simulink model "LCL_SIM"  (R2022a)
settings: Solver=VariableStepAuto  StartTime=0.0  StopTime=0.02*8  FixedStep=Ts  RelTol=1e-3
values from neighbouring files (symbols this model uses):
  C = 10e-06    (= 1e-05)    [LCL_Filter_Analysis.m]    (also in Lowpass_Filer_Design.m = tf(num_c,den_c,Ts); Parameter.m)
  L1 = 600e-06    (= 0.0006)    [LCL_Filter_Analysis.m]    (also in Lowpass_Filer_Design.m; Parameter.m)
  R = 2    [LCL_Filter_Analysis.m]    (also in Lowpass_Filer_Design.m = 1.5; Parameter.m = 1.5)
  Ts = 0.02/800    (= 2.5e-05)    [Lowpass_Filer_Design.m]    (also in Parameter.m)
  Vin = 360    [Parameter.m]
  Vtri = 3.05    [Parameter.m]
libraries: spsACVoltageSourceLib x9, spsIGBTDiodeLib x4, spsSeriesRLCBranchLib x3, spsCurrentMeasurementLib x3, spsVoltageMeasurementLib x2, spsDCVoltageSourceLib x1, spsGroundLib x1, simulink x1, slpidlib x1, spsTriangleGeneratorLib x1, spsPLLLib x1, spspowerguiLib x1
settings Model: Creator=hoang  LastModifiedBy=hoanghua
settings SolverCC: ZeroCrossAlgorithm=Adaptive  AlgebraicLoopSolver=TrustRegion
settings DataIOCC: ReturnWorkspaceOutputs=off
settings DebuggingCC: IgnoredZcDiagnostic=none  UnconnectedInputMsg=warning  UnconnectedOutputMsg=warning  UnconnectedLineMsg=warning  SFMachineParentedDataDiag=warning

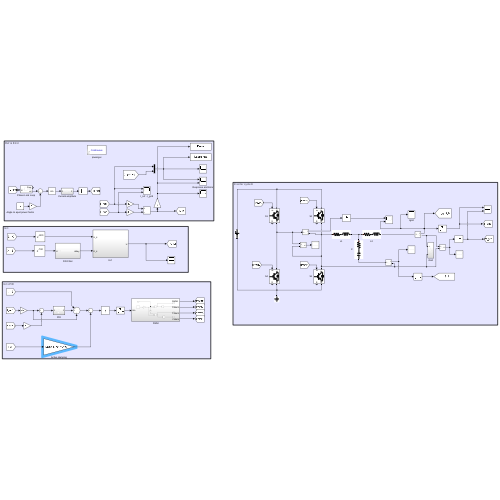
[thumbnail: Simulink's stored preview of the top-level diagram]
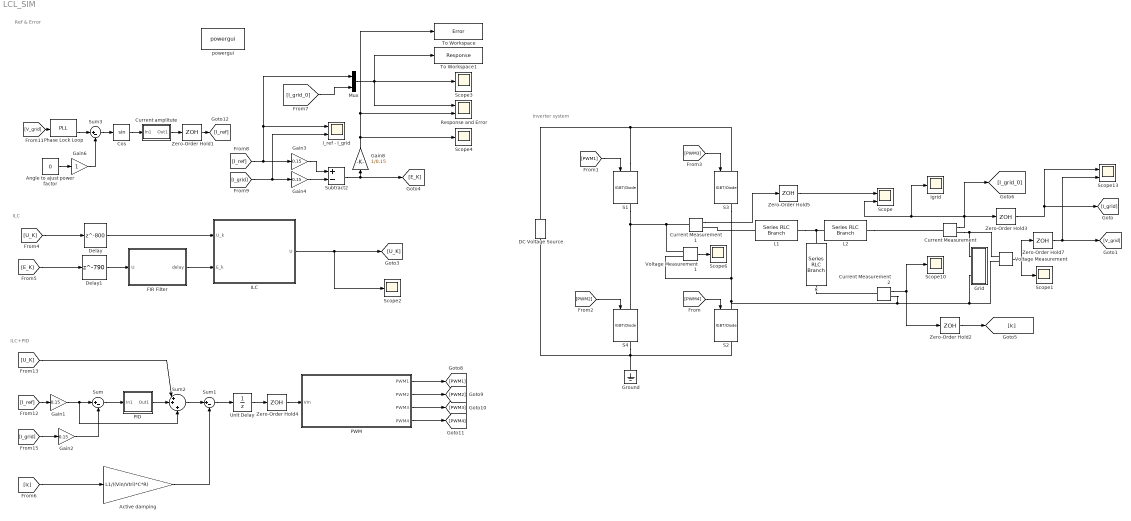
== system LCL_SIM ==
  note: ILC+PID
  note: Inverter system
  note: Ref & Error
  note: ILC
  Active damping : Gain  Gain=L1/((Vin/Vtri)*C*R)
  Angle to ajust power factor : Constant  Value=0
  C : spsSeriesRLCBranchLib/Series RLC Branch  LConnTagsString=__new0  RConnTagsString=__new0  BranchType=RC  Resistance=0.00  Inductance=600e-6  SetiL0=off  InitialCurrent=0  Capacitance=10e-6  Setx0=off  InitialVoltage=0  Measurements=None
  Cos : Trigonometry
  Current Measurement : spsCurrentMeasurementLib/Current Measurement  PhasorSimulation=off  OutputType=Complex  PSBequivalent=0
  Current Measurement1 : spsCurrentMeasurementLib/Current Measurement  PhasorSimulation=off  OutputType=Complex  PSBequivalent=0
  Current Measurement2 : spsCurrentMeasurementLib/Current Measurement  PhasorSimulation=off  OutputType=Magnitude  PSBequivalent=0
  Current amplitute : Subsystem
  DC Voltage Source : spsDCVoltageSourceLib/DC Voltage Source  Amplitude=360  Measurements=None
  Delay : Delay  DelayLength=800  SampleTime=Ts
  Delay1 : Delay  DelayLength=790  SampleTime=Ts
  FIR Filter : Subsystem
  Gain{1..4} (4 alike) : Gain  Gain=0.15
  Gain6 : Gain
  Gain8 : Gain  Gain=1/0.15
  Grid : Subsystem
  Ground : spsGroundLib/Ground  LConnTagsString=a
  "ILC " : Subsystem
  I_ref - I_grid : Scope  NumInputPorts=2
  Igrid : Scope
  L1 : spsSeriesRLCBranchLib/Series RLC Branch  LConnTagsString=__new0  RConnTagsString=__new0  BranchType=RL  Resistance=0  Inductance=600e-6  SetiL0=on  InitialCurrent=0  Capacitance=0  Setx0=off  InitialVoltage=0  Measurements=None
  L2 : spsSeriesRLCBranchLib/Series RLC Branch  LConnTagsString=__new0  RConnTagsString=__new0  BranchType=RL  Resistance=0  Inductance=150e-6  SetiL0=on  InitialCurrent=0  Capacitance=0  Setx0=off  InitialVoltage=0  Measurements=None
  Mux : Mux  Inputs=2
  PID : Subsystem
  PWM : Subsystem
  Phase Lock Loop : spsPLLLib/PLL  Fmin=45  Par_Init=[0, 50.1]  ParK=[180, 3200, 1]  TcD=1e-4  MaxRateChangeFreq=12  FilterCutOffFreq=25  Ts=0  AGC=on
      settings: SourceProductBaseCode=PS
  Response and Error : Scope  NumInputPorts=2
  S{1..4} (4 alike) : spsIGBTDiodeLib/IGBT//Diode  Ron=1e-3  Rs=1e5  Cs=inf  Measurements=on
  Scope : Scope  NumInputPorts=2
  Scope{1..4,6,10} (6 alike) : Scope
  Scope13 : Scope  NumInputPorts=2
  Subtract2 : Sum  Inputs=+-
  Sum : Sum  Inputs=|+-
  Sum1 : Sum  Inputs=|+-
  Sum2 : Sum  Inputs=|++|+
  Sum3 : Sum  Inputs=|+-
  To Workspace : ToWorkspace  VariableName=Error  SaveFormat=Timeseries  SampleTime=Ts
  To Workspace1 : ToWorkspace  VariableName=Response  SaveFormat=Timeseries  SampleTime=Ts
  Unit Delay : UnitDelay  SampleTime=-1  HasFrameUpgradeWarning=on
  Voltage Measurement : spsVoltageMeasurementLib/Voltage Measurement  PhasorSimulation=off  OutputType=Complex  PSBequivalent=0
  Voltage Measurement1 : spsVoltageMeasurementLib/Voltage Measurement  PhasorSimulation=off  OutputType=Complex  PSBequivalent=0
  Zero-Order Hold{1,3,5,7} (4 alike) : ZeroOrderHold  SampleTime=Ts
  Zero-Order Hold2 : ZeroOrderHold  SampleTime=Ts/100
  Zero-Order Hold4 : ZeroOrderHold  SampleTime=Ts/100
  powergui : spspowerguiLib/powergui  Priority=1  SimulationMode=Continuous  SampleTime=0.02/500  frequency=50  Iterations=50  frequencyindice=50  Pbase=100e6  ErrMax=1e-4  UnitsV=kV  UnitsW=MW  buscounter=0  FunctionMessages=on  echomessages=off  EnableUseOfTLC=off  CurrentSourceSwitches=off  DisableSnubberDevices=off  DisableRonSwitches=off  DisableVfSwitches=off  DisplayEquations=off  AutomaticDiscreteSolvers=off  SolverType=Tustin/Backward Euler (TBE)  Interpol=off  ExternalGateDelay=off  methode=off  Ts=100  x0status=blocks  SPID=off  SwTol=0  HookPort=off  NonlinearTolerance=1e-4  nMaxIteration=100  ContinueOnMaxIteration=off  RestoreLinks=warning  ResistiveCurrentMeasurement=off  Frange=[0:2:500]  Ylog=off  Xlog=on  ShowGrid=off  save=off  variable=ZData  structure=Igrid  ZoomFFT=off  StartTime=0.1  cycles=3  DisplayStyle=2  fundamental=50  FreqAxis=on  MaxFrequency=3000  frequencyindicesteady=1  RmsSteady=1  display=off
  wires:
  Gain4/1 -> Subtract2/2
  [E_K] -> Delay1/1
  [U_K] -> Delay/1
  [I_grid] -> I_ref - I_grid/2, Gain4/1
  Subtract2/1 -> Gain8/1, [E_K]
  "ILC "/1(U) -> [U_K], Scope2/1
  [I_ref] -> Mux/1, I_ref - I_grid/1, Gain3/1
  [V_grid] -> Phase Lock Loop/1
  [I_grid_0] -> Mux/2
  Mux/1 -> Scope3/1, To Workspace1/1, Response and Error/1
  Angle to ajust power factor/1 -> Gain6/1
  Phase Lock Loop/2 -> Sum3/1
  Gain6/1 -> Sum3/2
  Sum3/1 -> Cos/1
  Cos/1 -> Current amplitute/1(In1)
  Gain8/1 -> To Workspace/1, Response and Error/2, Scope4/1
  Gain3/1 -> Subtract2/1
  Delay/1 -> "ILC "/1(U_k)
  FIR Filter/1(delay) -> "ILC "/2(E_k)
  Delay1/1 -> FIR Filter/1(U)
  Current amplitute/1(Out1) -> Zero-Order Hold1/1
  Zero-Order Hold1/1 -> [I_ref]
  Voltage Measurement/1 -> Scope1/1, Zero-Order Hold7/1
  Current Measurement2/1 -> Zero-Order Hold2/1, Scope10/1
  [PWM2] -> S4/1
  Current Measurement1/1 -> Zero-Order Hold5/1
  Current Measurement/1 -> [I_grid_0], Igrid/1, Scope/2, Zero-Order Hold3/1
  [PWM3] -> S3/1
  Zero-Order Hold2/1 -> [Ic]
  Zero-Order Hold3/1 -> Scope13/1, [I_grid]
  Voltage Measurement1/1 -> Scope6/1
  Zero-Order Hold7/1 -> Scope13/2, [V_grid]
  [PWM1] -> S1/1
  Zero-Order Hold5/1 -> Scope/1
  [PWM4] -> S2/1
  PWM/1("PWM1 ") -> [PWM1]
  Zero-Order Hold4/1 -> PWM/1(Vm)
  PWM/4(PWM4) -> [PWM4]
  Active damping/1 -> Sum1/2
  Gain2/1 -> Sum/2
  [U_K] -> Sum2/1
  Sum/1 -> PID/1(In1)
  Sum1/1 -> Unit Delay/1
  Sum2/1 -> Sum1/1
  Unit Delay/1 -> Zero-Order Hold4/1
  PWM/3(PWM3) -> [PWM3]
  [I_ref] -> Gain1/1
  PWM/2(PWM2) -> [PWM2]
  [Ic] -> Active damping/1
  Gain1/1 -> Sum/1, Sum2/3
  [I_grid] -> Gain2/1
  PID/1(Out1) -> Sum2/2
  connections:
  C/RConn1 -- Current Measurement2/LConn1
  Current Measurement/RConn1 -- Voltage Measurement/LConn1 -- Grid/LConn1
  S1/LConn1 -- S3/LConn1 -- DC Voltage Source/RConn1
  S3/RConn1 -- Current Measurement2/RConn1 -- Voltage Measurement/LConn2 -- Grid/LConn2 -- S2/LConn1 -- Voltage Measurement1/LConn2
  DC Voltage Source/LConn1 -- S4/RConn1 -- S2/RConn1 -- Ground/LConn1
  Current Measurement1/LConn1 -- S4/LConn1 -- S1/RConn1 -- Voltage Measurement1/LConn1
  L1/LConn1 -- Current Measurement1/RConn1
  C/LConn1 -- L2/LConn1 -- L1/RConn1
  L2/RConn1 -- Current Measurement/LConn1

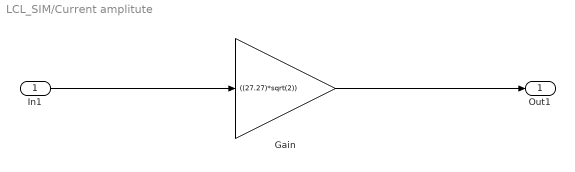
== system LCL_SIM/Current amplitute ==
  In1 : Inport
  Gain : Gain  Gain=((27.27)*sqrt(2))
  Out1 : Outport
  wires:
  In1/1 -> Gain/1
  Gain/1 -> Out1/1

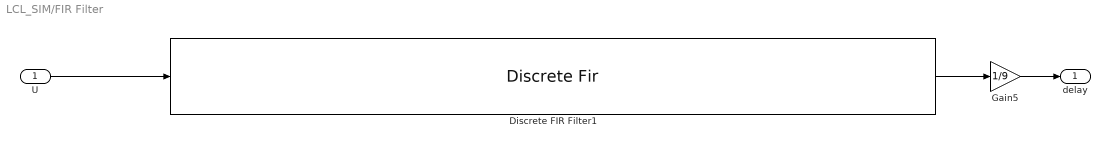
== system LCL_SIM/FIR Filter ==
  U : Inport
  Discrete FIR Filter1 : DiscreteFir  Coefficients=[1 1 1 1 1 1 1 1 1]  SampleTime=Ts
  Gain5 : Gain  Gain=1/9
  delay : Outport  VectorParamsAs1DForOutWhenUnconnected=off
  wires:
  Gain5/1 -> delay/1
  Discrete FIR Filter1/1 -> Gain5/1
  U/1 -> Discrete FIR Filter1/1

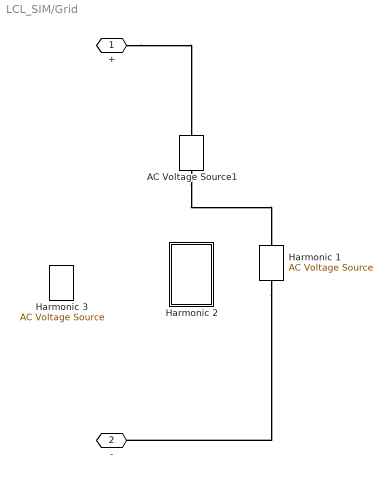
== system LCL_SIM/Grid ==
  AC Voltage Source1 : spsACVoltageSourceLib/AC Voltage Source  Amplitude=220*sqrt(2)  Phase=0  Frequency=50  SampleTime=0  Measurements=None  BusType=PV  Pref=6e3  Qref=0  Qmin=-inf  Qmax=+inf
  Harmonic 1 : spsACVoltageSourceLib/AC Voltage Source  Amplitude=220*sqrt(2)*0.01  Phase=0  Frequency=50*33  SampleTime=0  Measurements=None  BusType=PV  Pref=6e3  Qref=0  Qmin=-inf  Qmax=+inf
  Harmonic 2 : Subsystem
      settings: PortSchema="{\"entries\":[{\"content\":{\"sides\":[{\"content\":{\"connectorIds\":[]},\"type\":\"ConnectorPlacement.EquallySpacedRectSide\",\"uuid\":\"f60a8588-046c-4c4f-94c2-27eb35b2c768\"},{\"content\":{\"connectorIds\":[],\"side\":\"RIGHT\"},\"type\":\"ConnectorPlacement.EquallySpacedRectSide\",\"uuid\":\"a6fd0e6d-caa2-4954-9545-666586426112\"},{\"content\":{\"connectorIds\":[\"LConn1\"],\"side\":\"TOP\"},\"type\":\"ConnectorPlacement.EquallySpacedRectSide\",\"uuid\":\"3887d386-67a4-4090-b26b-c77f8cd89017\"},{\"content\":{\"connectorIds\":[\"RConn1\"],\"side\":\"BOTTOM\"},\"type\":\"ConnectorPlacement.EquallySpacedRectSide\",\"uuid\":\"506826a6-9c45-4d5d-96d6-c56dbc9a3480\"}]},\"type\":\"ConnectorPlacement.EquallySpacedConnector\",\"uuid\":\"c15ad883-a9a3-491e-b546-5f76a0de8772\"}],\"packageUris\":[\"http://schema.mathworks.com/mf0/Connector/19700101\"],\"version\":\"1.0\"}"
  Harmonic 3 : spsACVoltageSourceLib/AC Voltage Source  Amplitude=220*sqrt(2)*0.1  Phase=0  Frequency=50*3  SampleTime=0  Measurements=None  BusType=PV  Pref=6e3  Qref=0  Qmin=-inf  Qmax=+inf
  + : PMIOPort  Side=Left
  - : PMIOPort  Port=2  Side=Left
  connections:
  +/RConn1 -- AC Voltage Source1/RConn1
  AC Voltage Source1/LConn1 -- Harmonic 1/RConn1
  Harmonic 1/LConn1 -- -/RConn1

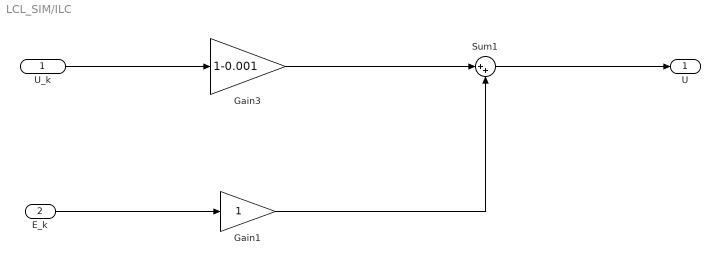
== system LCL_SIM/ILC  ==
  U_k : Inport
  E_k : Inport  Port=2
  Gain1 : Gain
  Gain3 : Gain  Gain=1-0.001
  Sum1 : Sum  Inputs=|++
  U : Outport  VectorParamsAs1DForOutWhenUnconnected=off
  wires:
  U_k/1 -> Gain3/1
  Sum1/1 -> U/1
  E_k/1 -> Gain1/1
  Gain3/1 -> Sum1/1
  Gain1/1 -> Sum1/2

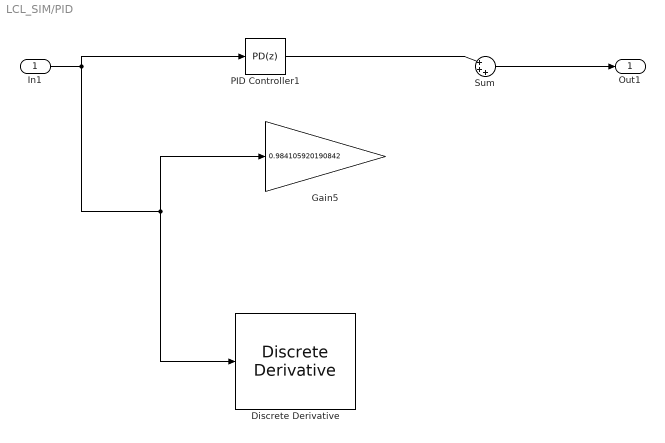
== system LCL_SIM/PID ==
  In1 : Inport
  Discrete Derivative : simulink/Discrete/Discrete Derivative  gainval=6.59449920156203e-05  ICPrevScaledInput=0.0  OutMin=[]  OutMax=[]  OutDataType=fixdt(1, 16)  OutScaling=2^-10  DoSatur=off
  Gain5 : Gain  Gain=0.984105920190842
  PID Controller1 : slpidlib/PID Controller  Controller=PD  Form=Parallel  TimeDomain=Discrete-time  UseExternalTs=off  SampleTime=Ts  IntegratorMethod=Forward Euler  FilterMethod=Forward Euler  ControllerParametersSource=internal  P=0.984105920190842  I=2200  UseKiTs=off  D=6.59449920156203e-05  N=10000000000000000  UseFilter=off  TunerSelectOption=Transfer Function Based (PID Tuner App)  InitialConditionSource=internal  InitialConditionForIntegrator=0  InitialConditionForFilter=0  DifferentiatorICPrevScaledInput=0  ExternalReset=none  TrackingMode=off  Kt=1  LimitOutput=off  SatLimitsSource=internal  UpperSaturationLimit=inf  LowerSaturationLimit=-inf  LinearizeAsGain=on  AntiWindupMode=none  Kb=1  POutMin=[]  POutMax=[]  IOutMin=[]  IOutMax=[]  DOutMin=[]  DOutMax=[]  NOutMin=[]  NOutMax=[]  SumOutMin=[]  SumOutMax=[]  SaturationOutMin=[]  SaturationOutMax=[]  PParamMin=[]  PParamMax=[]  IParamMin=[]  IParamMax=[]  DParamMin=[]  DParamMax=[]  NParamMin=[]  NParamMax=[]  KbParamMin=[]  KbParamMax=[]  KtParamMin=[]  KtParamMax=[]  KbOutMin=[]  KbOutMax=[]  KtOutMin=[]  KtOutMax=[]  IntegratorOutMin=[]  IntegratorOutMax=[]  FilterOutMin=[]  FilterOutMax=[]  SumI1OutMin=[]  SumI1OutMax=[]  SumI2OutMin=[]  SumI2OutMax=[]  SumI3OutMin=[]  SumI3OutMax=[]  SumI4OutMin=[]  SumI4OutMax=[]  SumDOutMin=[]  SumDOutMax=[]  DifferentiatorOutMin=[]  DifferentiatorOutMax=[]  FilterDiffOutCoefMin=[]  FilterDiffOutCoefMax=[]  ReciprocalOutMin=[]  ReciprocalOutMax=[]  SumDenOutMin=[]  SumDenOutMax=[]  SumNumOutMin=[]  SumNumOutMax=[]  DivideOutMin=[]  DivideOutMax=[]  UdiffTsProdOutMin=[]  UdiffTsProdOutMax=[]  NTsProdOutMin=[]  NTsProdOutMax=[]  UintegralTsProdOutMin=[]  UintegralTsProdOutMax=[]  UngainTsProdOutMin=[]  UngainTsProdOutMax=[]  IntegratorContinuousStateAttributes=''  IntegratorStateMustResolveToSignalObject=off  IntegratorRTWStateStorageClass=Auto  FilterContinuousStateAttributes=''  FilterStateMustResolveToSignalObject=off  FilterRTWStateStorageClass=Auto  ParallelPVariant=InternalParameters  IdealPVariant=Disabled  IVariant=Disabled  DVariant=InternalParameters  IntegratorVariant=Disabled  SatVariant=Disabled  AWVariant=Disabled  PCopyVariant=Disabled  TRVariant=Disabled  FdbkBlocksVariant=Forward  IdealPFdbkVariant=Disabled  SatFdbkVariant=Disabled  DerivativeFilterVariant=Differentiator  NVariant=Passthrough  NCopyVariant=Disabled_SignalSpec  FilterICVariant=InternalICsDifferentiator  IntegratorICVariant=Disabled  ExternalResetVariant=Disabled  TRSumVariant=Passthrough  SumFdbkVariant=Disabled  SumVariant=Sum_PD  TsampFilterVariant=InternalTs  TsampNgainVariant=Passthrough  TsampIntegralVariant=Disabled_SignalSpec  ExternalSaturationOutDataTypeStr=Inherit: Same as second input  aMode=0
  Sum : Sum  Inputs=|+++
  Out1 : Outport  VectorParamsAs1DForOutWhenUnconnected=off
  wires:
  Sum/1 -> Out1/1
  In1/1 -> PID Controller1/1, Discrete Derivative/1, Gain5/1
  PID Controller1/1 -> Sum/1

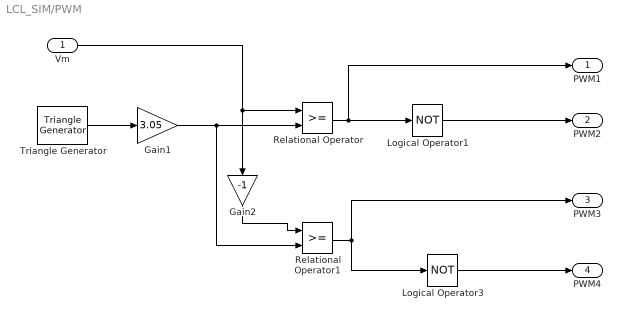
== system LCL_SIM/PWM ==
  Vm : Inport
  Gain1 : Gain  Gain=3.05
  Gain2 : Gain  Gain=-1
  Logical Operator1 : Logic  Operator=NOT  AllPortsSameDT=off  OutDataTypeStr=boolean
  Logical Operator3 : Logic  Operator=NOT  AllPortsSameDT=off  OutDataTypeStr=boolean
  Relational Operator : RelationalOperator  OutDataTypeStr=boolean  RndMeth=Simplest  InputSameDT=off
  Relational Operator1 : RelationalOperator  OutDataTypeStr=boolean  RndMeth=Simplest  InputSameDT=off
  Triangle Generator : spsTriangleGeneratorLib/Triangle Generator  Freq=10e3  Phase=0  Ts=0
  "PWM1 " : Outport  VectorParamsAs1DForOutWhenUnconnected=off
  PWM2 : Outport  Port=2  VectorParamsAs1DForOutWhenUnconnected=off
  PWM3 : Outport  Port=3  VectorParamsAs1DForOutWhenUnconnected=off
  PWM4 : Outport  Port=4  VectorParamsAs1DForOutWhenUnconnected=off
  wires:
  Vm/1 -> Gain2/1, Relational Operator/1
  Triangle Generator/1 -> Gain1/1
  Gain1/1 -> Relational Operator1/2, Relational Operator/2
  Relational Operator/1 -> "PWM1 "/1, Logical Operator1/1
  Logical Operator1/1 -> PWM2/1
  Relational Operator1/1 -> PWM3/1, Logical Operator3/1
  Gain2/1 -> Relational Operator1/1
  Logical Operator3/1 -> PWM4/1

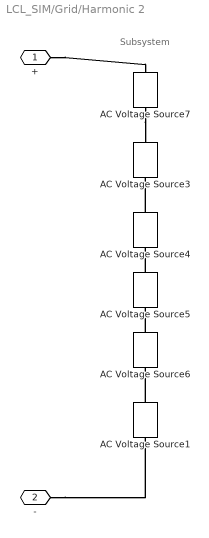
== system LCL_SIM/Grid/Harmonic 2 ==
  note: Subsystem
  AC Voltage Source1 : spsACVoltageSourceLib/AC Voltage Source  Amplitude=220*sqrt(2)*0.02  Phase=0  Frequency=50*13  SampleTime=0  Measurements=None  BusType=PV  Pref=6e3  Qref=0  Qmin=-inf  Qmax=+inf
  AC Voltage Source3 : spsACVoltageSourceLib/AC Voltage Source  Amplitude=220*sqrt(2)*0.05  Phase=90  Frequency=50*5  SampleTime=0  Measurements=None  BusType=PV  Pref=6e3  Qref=0  Qmin=-inf  Qmax=+inf
  AC Voltage Source4 : spsACVoltageSourceLib/AC Voltage Source  Amplitude=220*sqrt(2)*0.03  Phase=0  Frequency=50*7  SampleTime=0  Measurements=None  BusType=PV  Pref=6e3  Qref=0  Qmin=-inf  Qmax=+inf
  AC Voltage Source5 : spsACVoltageSourceLib/AC Voltage Source  Amplitude=220*sqrt(2)*0.03  Phase=0  Frequency=50*9  SampleTime=0  Measurements=None  BusType=PV  Pref=6e3  Qref=0  Qmin=-inf  Qmax=+inf
  AC Voltage Source6 : spsACVoltageSourceLib/AC Voltage Source  Amplitude=220*sqrt(2)*0.02  Phase=0  Frequency=50*11  SampleTime=0  Measurements=None  BusType=PV  Pref=6e3  Qref=0  Qmin=-inf  Qmax=+inf
  AC Voltage Source7 : spsACVoltageSourceLib/AC Voltage Source  Amplitude=220*sqrt(2)*0.1  Phase=0  Frequency=50*3  SampleTime=0  Measurements=None  BusType=PV  Pref=6e3  Qref=0  Qmin=-inf  Qmax=+inf
  + : PMIOPort  Side=Left
  - : PMIOPort  Port=2  Side=Right
  connections:
  AC Voltage Source7/LConn1 -- AC Voltage Source3/RConn1
  AC Voltage Source5/RConn1 -- AC Voltage Source4/LConn1
  AC Voltage Source4/RConn1 -- AC Voltage Source3/LConn1
  AC Voltage Source1/RConn1 -- AC Voltage Source6/LConn1
  +/RConn1 -- AC Voltage Source7/RConn1
  AC Voltage Source6/RConn1 -- AC Voltage Source5/LConn1
  -/RConn1 -- AC Voltage Source1/LConn1
